simulink model "quad_control_sim_q"  (R2013a)
settings: Solver=ode3  StartTime=0.0  StopTime=5  FixedStep=0.005  RelTol=1e-3
values from neighbouring files (symbols this model uses):
  initial_states = [0;0;0;0;0;0;q0_init;0;q1_init;0;q2_init;0;q3_init;0]    [quad_control_sim_script_q.m]
  inputs = [x_accel_ref; y_accel_ref; a_u]    [quad_control_sim_script_q.m]
  params = [m;g;l;Jxx;Jyy;Jzz;k1;k2;k3;k4;b1;b2;b3;b4; d]    [quad_control_sim_script_q.m]
  pq = 1.2    [quad_control_sim_script_q.m]
  pw = 18    [quad_control_sim_script_q.m]
settings Model: Creator=Ken Katagiri  LastModifiedBy=Ken Katagiri

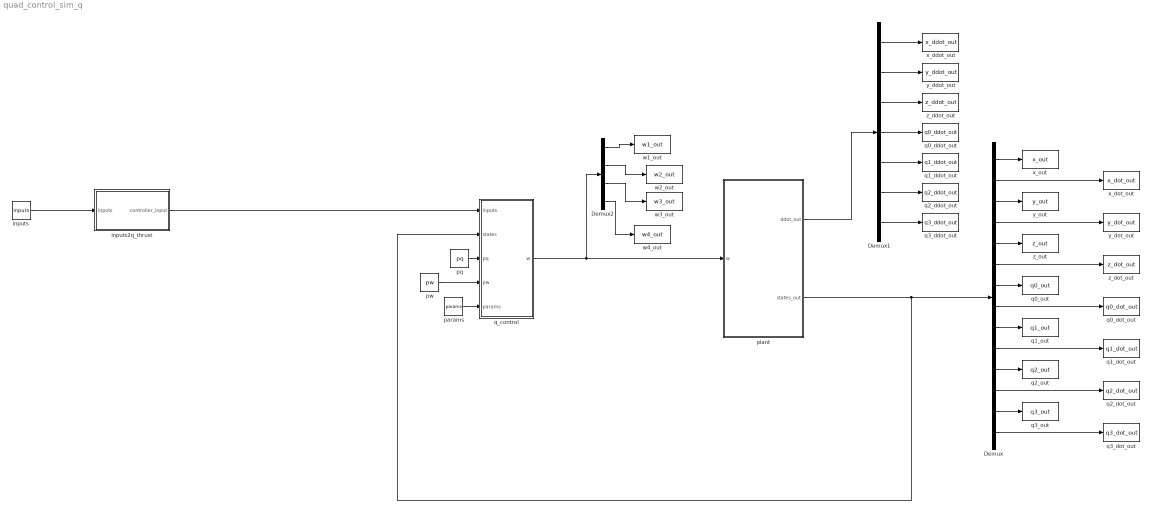
== system quad_control_sim_q ==
  Demux : Demux  Outputs=14
  Demux1 : Demux  Outputs=7
  Demux2 : Demux
  inputs : Constant  Value=inputs
  inputs2q_thrust : MATLAB Function  TreatAsAtomicUnit=on
  params : Constant  Value=params
  plant : Subsystem
  pq : Constant  Value=pq
  pw : Constant  Value=pw
  q0_ddot_out : ToWorkspace  VariableName=q0_ddot_out  SampleTime=-1
  q0_dot_out : ToWorkspace  VariableName=q0_dot_out  SampleTime=-1
  q0_out : ToWorkspace  VariableName=q0_out  SampleTime=-1
  q1_ddot_out : ToWorkspace  VariableName=q1_ddot_out  SampleTime=-1
  q1_dot_out : ToWorkspace  VariableName=q1_dot_out  SampleTime=-1
  q1_out : ToWorkspace  VariableName=q1_out  SampleTime=-1
  q2_ddot_out : ToWorkspace  VariableName=q2_ddot_out  SampleTime=-1
  q2_dot_out : ToWorkspace  VariableName=q2_dot_out  SampleTime=-1
  q2_out : ToWorkspace  VariableName=q2_out  SampleTime=-1
  q3_ddot_out : ToWorkspace  VariableName=q3_ddot_out  SampleTime=-1
  q3_dot_out : ToWorkspace  VariableName=q3_dot_out  SampleTime=-1
  q3_out : ToWorkspace  VariableName=q3_out  SampleTime=-1
  q_control : MATLAB Function  TreatAsAtomicUnit=on
  w1_out : ToWorkspace  VariableName=w1_out  SampleTime=-1
  w2_out : ToWorkspace  VariableName=w2_out  SampleTime=-1
  w3_out : ToWorkspace  VariableName=w3_out  SampleTime=-1
  w4_out : ToWorkspace  VariableName=w4_out  SampleTime=-1
  x_ddot_out : ToWorkspace  VariableName=x_ddot_out  SampleTime=-1
  x_dot_out : ToWorkspace  VariableName=x_dot_out  SampleTime=-1
  x_out : ToWorkspace  VariableName=x_out  SampleTime=-1
  y_ddot_out : ToWorkspace  VariableName=y_ddot_out  SampleTime=-1
  y_dot_out : ToWorkspace  VariableName=y_dot_out  SampleTime=-1
  y_out : ToWorkspace  VariableName=y_out  SampleTime=-1
  z_ddot_out : ToWorkspace  VariableName=z_ddot_out  SampleTime=-1
  z_dot_out : ToWorkspace  VariableName=z_dot_out  SampleTime=-1
  z_out : ToWorkspace  VariableName=z_out  SampleTime=-1
  wires:
  Demux/1 -> x_out/1
  Demux/3 -> y_out/1
  Demux/5 -> z_out/1
  Demux/7 -> q0_out/1
  Demux/9 -> q1_out/1
  Demux/11 -> q2_out/1
  Demux/13 -> q3_out/1
  Demux/2 -> x_dot_out/1
  Demux/4 -> y_dot_out/1
  Demux/6 -> z_dot_out/1
  Demux/8 -> q0_dot_out/1
  Demux/10 -> q1_dot_out/1
  Demux/12 -> q2_dot_out/1
  Demux/14 -> q3_dot_out/1
  Demux1/1 -> x_ddot_out/1
  Demux1/2 -> y_ddot_out/1
  Demux1/3 -> z_ddot_out/1
  Demux1/4 -> q0_ddot_out/1
  Demux1/5 -> q1_ddot_out/1
  Demux1/6 -> q2_ddot_out/1
  Demux1/7 -> q3_ddot_out/1
  plant/1(ddot_out) -> Demux1/1
  params/1 -> q_control/5(params)
  pq/1 -> q_control/3(pq)
  plant/2(states_out) -> q_control/2(states), Demux/1
  pw/1 -> q_control/4(pw)
  inputs/1 -> inputs2q_thrust/1(inputs)
  inputs2q_thrust/1(controller_input) -> q_control/1(inputs)
  q_control/1(w) -> Demux2/1, plant/1(w)
  Demux2/1 -> w1_out/1
  Demux2/2 -> w2_out/1
  Demux2/3 -> w3_out/1
  Demux2/4 -> w4_out/1

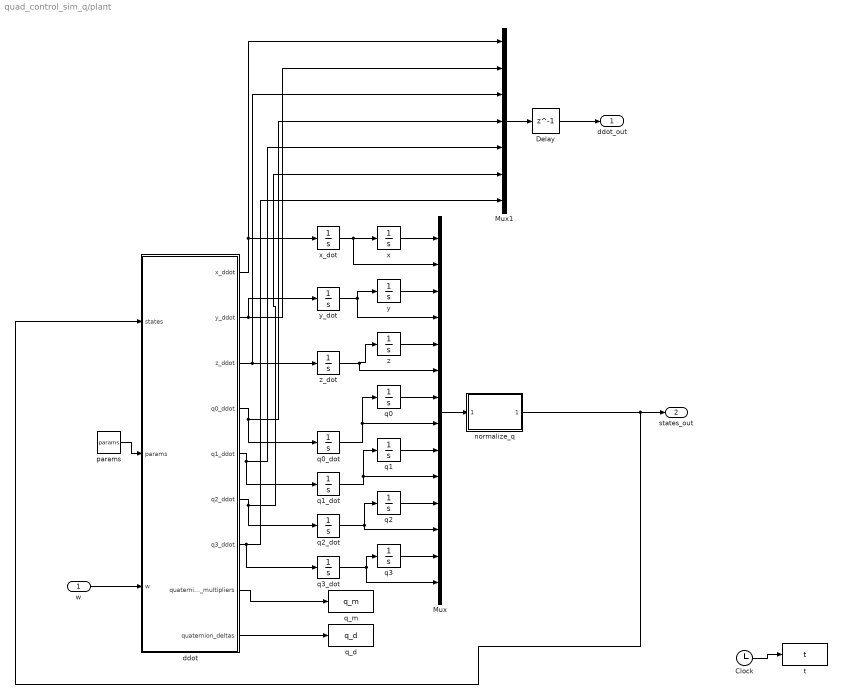
== system quad_control_sim_q/plant ==
  w : Inport
  Clock : Clock
  Delay : Delay  DelayLength=1  InitialCondition=[0; 0; 0; 0; 0; 0; 0]
  Mux : Mux  Inputs=14
  Mux1 : Mux  Inputs=7
  ddot : MATLAB Function  TreatAsAtomicUnit=on
  normalize_q : MATLAB Function  TreatAsAtomicUnit=on
  params : Constant  Value=params
  q0 : Integrator  InitialCondition=initial_states(7)
  q0_dot : Integrator
  q1 : Integrator  InitialCondition=initial_states(9)
  q1_dot : Integrator
  q2 : Integrator  InitialCondition=initial_states(11)
  q2_dot : Integrator
  q3 : Integrator  InitialCondition=initial_states(13)
  q3_dot : Integrator
  q_d : ToWorkspace  VariableName=q_d  SampleTime=-1
  q_m : ToWorkspace  VariableName=q_m  SampleTime=-1
  t : ToWorkspace  VariableName=t  SampleTime=-1
  x : Integrator  InitialCondition=initial_states(1)
  x_dot : Integrator
  y : Integrator  InitialCondition=initial_states(2)
  y_dot : Integrator
  z : Integrator  InitialCondition=initial_states(3)
  z_dot : Integrator
  ddot_out : Outport
  states_out : Outport  Port=2
  wires:
  ddot/7(q3_ddot) -> q3_dot/1, Mux1/7
  ddot/6(q2_ddot) -> Mux1/6, q2_dot/1
  ddot/5(q1_ddot) -> Mux1/5, q1_dot/1
  ddot/1(x_ddot) -> Mux1/1, x_dot/1
  ddot/2(y_ddot) -> Mux1/2, y_dot/1
  ddot/3(z_ddot) -> Mux1/3, z_dot/1
  ddot/4(q0_ddot) -> Mux1/4, q0_dot/1
  x_dot/1 -> Mux/2, x/1
  y_dot/1 -> Mux/4, y/1
  q3_dot/1 -> Mux/14, q3/1
  q2_dot/1 -> Mux/12, q2/1
  q1_dot/1 -> Mux/10, q1/1
  q0_dot/1 -> Mux/8, q0/1
  x/1 -> Mux/1
  y/1 -> Mux/3
  z/1 -> Mux/5
  z_dot/1 -> Mux/6, z/1
  q0/1 -> Mux/7
  q1/1 -> Mux/9
  q2/1 -> Mux/11
  q3/1 -> Mux/13
  params/1 -> ddot/2(params)
  Clock/1 -> t/1
  w/1 -> ddot/3(w)
  ddot/8(quaternion_multipliers) -> q_m/1
  ddot/9(quaternion_deltas) -> q_d/1
  Mux/1 -> normalize_q/1(states_in)
  normalize_q/1(states_out) -> states_out/1, ddot/1(states)
  Mux1/1 -> Delay/1
  Delay/1 -> ddot_out/1

== matlab function quad_control_sim_q/plant/normalize_q ==
  data: states_in input size=14; states_out output
function states_out = fcn(states_in)
%#codegen
    q0_in = states_in(7); q1_in = states_in(9); q2_in = states_in(11); q3_in = states_in(13);
    q_norm = norm([q0_in, q1_in, q2_in, q3_in]);
    q0_out = q0_in/q_norm; q1_out = q1_in/q_norm; q2_out = q2_in/q_norm; q3_out = q3_in/q_norm; 
    states_out = [states_in(1); states_in(2); states_in(3); states_in(4); states_in(5); states_in(6); ...
            q0_out; states_in(8); q1_out; states_in(10); q2_out; states_in(12); q3_out; states_in(14)];

== matlab function quad_control_sim_q/plant/ddot ==
  data: states input size=14; x_ddot output; y_ddot output; z_ddot output; q0_ddot output; q1_ddot output; q2_ddot output; q3_ddot output; params input; w input; quaternion_multipliers output; quaternion_deltas output
function [x_ddot, y_ddot, z_ddot, q0_ddot, q1_ddot, q2_ddot, q3_ddot, quaternion_multipliers, quaternion_deltas]= ddot(states, params, w)
%#codegen    
    m=params(1);
    g=params(2);
    l=params(3);

    Jxx=params(4);
    Jyy=params(5);
    Jzz=params(6);

    k1 = params(7);
    k2 = params(8);
    k3 = params(9);
    k4 = params(10);

    b1 = params(11);
    b2 = params(12);
    b3 = params(13);
    b4 = params(14);
    
    d = params(15);

    w1 = w(1);
    w2 = w(2);
    w3 = w(3);
    w4 = w(4);
    
    x = states(1); x_dot = states(2); y = states(3); y_dot = states(4); z = states(5); z_dot = states(6);

    q0 = states(7); q0_dot = states(8); q1 = states(9); q1_dot = states(10);
    q2 = states(11); q2_dot = states(12); q3 = states(13); q3_dot = states(14);
    
    upphi_x = 2*(k1*w1^2+k2*w2^2+k3*w3^2+k4*w4^2)*(q2*q0+q1*q3) ...
                + (-b1*w1^2+b2*w2^2+b3*w3^2-b4*w4^2)*(1-2*(q2^2+q3^2)) ...
                + 2*(b1*w1^2+b2*w2^2-b3*w3^2-b4*w4^2)*(q1*q2-q3*q0) - d*x_dot;
            
    upphi_y = 2*(k1*w1^2+k2*w2^2+k3*w3^2+k4*w4^2)*(q3*q2-q1*q0) ...
                + 2*(-b1*w1^2+b2*w2^2+b3*w3^2-b4*w4^2)*(q3*q0+q1*q2) ...
                + (b1*w1^2+b2*w2^2-b3*w3^2-b4*w4^2)*(1-2*(q1^2+q3^2)) - d*y_dot;
            
    upphi_z = (k1*w1^2+k2*w2^2+k3*w3^2+k4*w4^2)*(1-2*(q1^2+q2^2)) ...
                + 2*(-b1*w1^2+b2*w2^2+b3*w3^2-b4*w4^2)*(q3*q1-q2*q0) ...
                + 2*(b1*w1^2+b2*w2^2-b3*w3^2-b4*w4^2)*(q1*q0+q3*q2) - d*z_dot;
            
    T_e2E = [1-2*(q2^2+q3^2), 2*(q1*q2-q3*q0), 2*(q2*q0+q1*q3);
            2*(q3*q0+q1*q2), 1-2*(q1^2+q3^2), 2*(q3*q2-q1*q0);
            2*(q3*q1-q2*q0), 2*(q1*q0+q3*q2), 1-2*(q1^2+q2^2)];

            
    force_mult_1 = [-b1*w1^2-b3*w3^2; b1*w1^2+b3*w3^2; k1*w1^2-k3*w3^2];
    force_mult_2 = [b2*w2^2+b4*w4^2; b2*w2^2+b4*w4^2; k2*w2^2-k4*w4^2];
        
    force_mult_1_E = T_e2E*force_mult_1;
    force_mult_2_E = T_e2E*force_mult_2;
        
    dx1_dq0 = (l/sqrt(2))*[-2*q3; 2*q3; 2*q1-2*q2];
    dx2_dq0 = (l/sqrt(2))*[-2*q3; -2*q3; 2*q1+2*q2];
    upphi_q0 = dot(force_mult_1_E, dx1_dq0) + dot(force_mult_2_E, dx2_dq0);
    
    dx1_dq1 = (l/sqrt(2))*[2*q2; 2*q2-4*q1; 2*q0+2*q3];
    dx2_dq1 = (l/sqrt(2))*[2*q2; -4*q1-2*q2; 2*q0-2*q3];
    upphi_q1 = dot(force_mult_1_E, dx1_dq1) + dot(force_mult_2_E, dx2_dq1);
        
    dx1_dq2 = (l/sqrt(2))*[2*q1-4*q2; 2*q1; 2*q3-2*q0];
    dx2_dq2 = (l/sqrt(2))*[2*q1+4*q2; -2*q1; 2*q3+2*q0];
    upphi_q2 = dot(force_mult_1_E, dx1_dq2) + dot(force_mult_2_E, dx2_dq2);
    
    dx1_dq3 = (l/sqrt(2))*[-2*q0-4*q3; 2*q0-4*q3; 2*q1+2*q2];
    dx2_dq3 = (l/sqrt(2))*[-2*q0+4*q3; -4*q3-2*q0; 2*q2-2*q1];
    upphi_q3 = dot(force_mult_1_E, dx1_dq3) + dot(force_mult_2_E, dx2_dq3);
    
        
    delta1 = upphi_x;

    delta2 = upphi_y;

    delta3 = upphi_z;


    delta4 = upphi_q0 ...
                -8*Jxx*q0_dot*q1_dot*q1-8*Jyy*q0_dot*q2_dot*q2-8*Jzz*q0_dot*q3_dot*q3 ...
                +8*Jxx*q1_dot^2*q0+8*Jyy*q2_dot^2*q0+8*Jzz*q3_dot^2*q0 ...
                +(8*Jxx-8*Jyy)*q1_dot*q2_dot*q3+(8*Jzz-8*Jxx)*q1_dot*q3_dot*q2+(8*Jyy-8*Jzz)*q2_dot*q3_dot*q1;

    delta5 = upphi_q1 ...
                -8*Jxx*q0_dot*q1_dot*q0-8*Jyy*q1_dot*q3_dot*q3-8*Jzz*q1_dot*q2_dot*q2 ...
                +(8*Jyy-8*Jzz)*q2_dot*q3_dot*q0+(8*Jxx-8*Jyy)*q0_dot*q3_dot*q2+(8*Jzz-8*Jxx)*q0_dot*q2_dot*q3 ...
                +8*Jxx*q0_dot^2*q1+8*Jyy*q3_dot^2*q1+8*Jzz*q2_dot^2*q1;

    delta6 = upphi_q2 ...
                -8*Jxx*q2_dot*q3_dot*q3-8*Jyy*q0_dot*q2_dot*q0-8*Jzz*q1_dot*q2_dot*q1 ...
                +8*Jxx*q3_dot^2*q2+8*Jyy*q0_dot^2*q2+8*Jzz*q1_dot^2*q2 ...
                +8*(Jxx-Jyy)*q0_dot*q3_dot*q1+8*(Jyy-Jzz)*q0_dot*q1_dot*q3+8*(Jzz-Jxx)*q1_dot*q3_dot*q0;

    delta7 = upphi_q3 ...
                -8*Jxx*q2_dot*q3_dot*q2-8*Jyy*q1_dot*q3_dot*q1-8*Jzz*q0_dot*q3_dot*q0 ...
                +8*Jxx*q2_dot^2*q3+8*Jyy*q1_dot^2*q3+8*Jzz*q0_dot^2*q3 ...
                +(8*Jzz-8*Jxx)*q0_dot*q2_dot*q1+(8*Jxx-8*Jyy)*q1_dot*q2_dot*q0+(8*Jyy-8*Jzz)*q0_dot*q1_dot*q2;
            

    quaternion_deltas = [delta4; delta5; delta6; delta7; -q0_dot^2-q1_dot^2-q2_dot^2-q3_dot^2];

    quaternion_multipliers = ...
        [4*Jxx*q1^2+4*Jyy*q2^2+4*Jzz*q3^2, -4*Jzz*q2*q3+4*Jyy*q2*q3-4*Jxx*q0*q1, -4*Jxx*q1*q3+4*Jzz*q1*q3-4*Jyy*q0*q2, -4*Jyy*q1*q2+4*Jxx*q1*q2-4*Jzz*q0*q3;
         -4*Jzz*q2*q3+4*Jyy*q2*q3-4*Jxx*q0*q1, 4*Jxx*q0^2+4*Jyy*q3^2+4*Jzz*q2^2, -4*Jyy*q0*q3+4*Jxx*q0*q3-4*Jzz*q1*q2, -4*Jxx*q0*q2+4*Jzz*q0*q2-4*Jyy*q1*q3;
         -4*Jxx*q1*q3+4*Jzz*q1*q3-4*Jyy*q0*q2, -4*Jyy*q0*q3+4*Jxx*q0*q3-4*Jzz*q1*q2, 4*Jxx*q3^2+4*Jyy*q0^2+4*Jzz*q1^2, -4*Jzz*q0*q1+4*Jyy*q0*q1-4*Jxx*q2*q3;
         -4*Jyy*q1*q2+4*Jxx*q1*q2-4*Jzz*q0*q3, -4*Jxx*q0*q2+4*Jzz*q0*q2-4*Jyy*q1*q3, -4*Jzz*q0*q1+4*Jyy*q0*q1-4*Jxx*q2*q3, 4*Jxx*q2^2+4*Jyy*q1^2+4*Jzz*q0^2;
         q0, q1, q2, q3];

    q_ddot = quaternion_multipliers\quaternion_deltas;

    
    
    
    x_ddot = delta1/m;
    y_ddot = delta2/m;
    z_ddot= delta3/m-g;  
    q0_ddot = q_ddot(1);
    q1_ddot = q_ddot(2);
    q2_ddot = q_ddot(3);
    q3_ddot = q_ddot(4);

== matlab function quad_control_sim_q/q_control ==
  data: inputs input; states input; w output size=4; pq input; pw input; params input
function w = fcn(inputs, states, pq, pw, params)

    m=params(1);
    g=params(2);
    l=params(3);

    Jxx=params(4);
    Jyy=params(5);
    Jzz=params(6);

    k1 = params(7);
    k2 = params(8);
    k3 = params(9);
    k4 = params(10);

    b1 = params(11);
    b2 = params(12);
    b3 = params(13);
    b4 = params(14);
    
    d = params(15);
    
    q0=states(7); q1=states(9); q2=states(11); q3=states(13);
    q0_dot=states(8); q1_dot=states(10); q2_dot=states(12); q3_dot=states(14);

    q0_r = inputs(1); q1_r = inputs(2); q2_r = inputs(3); q3_r = inputs(4); a_u = inputs(5);
    
    q0_err = q0_r*q0+q1_r*q1+q2_r*q2+q3_r*q3;
    q1_err = q1_r*q0+q3_r*q2-q0_r*q1-q3_r*q3;
    q2_err = q2_r*q0+q1_r*q3-q3_r*q1-q0_r*q2;
    q3_err = q3_r*q0+q2_r*q1-q1_r*q2-q0_r*q3;
    
    if q0_err < 0
        q1_err = -q1_err;
        q2_err = -q2_err;
        q3_err = -q3_err;
    end

    %%%%%%%%%%%%NORMALIZE ERROR QUATERNION
    n = norm([q0_err; q1_err; q2_err; q3_err]);
    q0_err = q0_err/n; q1_err = q1_err/n; q2_err = q2_err/n; q3_err = q3_err/n; 
    
    wx = 2*(q1_dot*q0+q2_dot*q3-q3_dot*q2-q0_dot*q1);
    wy = 2*(q3_dot*q1+q2_dot*q0-q1_dot*q3-q0_dot*q2);
    wz = 2*(q3_dot*q0+q1_dot*q2-q2_dot*q1-q0_dot*q3);
    
    
    %disp('------------');

    tau_x = pq*q1_err-pw*Jxx*(l/sqrt(2))*wx;
    tau_y = pq*q2_err-pw*Jyy*(l/sqrt(2))*wy;
    tau_z = pq*q3_err-pw*Jzz*l*(wz);

    gamma1 = (sqrt(2)/l)*tau_x;
    gamma2 = (sqrt(2)/l)*tau_y;
    gamma3 = (m*a_u)/(cos(2*acos(q0)));
    gamma4 = (1/l)*tau_z;
    

    w3_sq3 = (gamma4+(b1/k1)*((gamma2-gamma1)/2)+(b2/k2)*((gamma2+gamma3)/2)+(b4/k4)*((gamma3-gamma1)/2))/((b1/k1)*k3+(b2/k2)*k3+b3+(b4/k4)*k3);
    w1_sq3 = ((gamma1-gamma2)/2+k3*w3_sq3)/k1;
    w2_sq3 = ((gamma2+gamma3)/2-k3*w3_sq3)/k2;
    w4_sq3 = ((gamma3-gamma1)/2-k3*w3_sq3)/k4;
    
    w2_sq = ((b1/k1)*((gamma1+gamma3)/2)+(b3/k3)*((gamma2+gamma3)/2)+(b4/k4)*((gamma1+gamma2)/2)-gamma4)/((b1/k1)*k2+b2+(b3/k3)*k2+(b4/k4)*k2);
    w1_sq = ((gamma1+gamma3)/2-k2*w2_sq)/k1;
    w3_sq = ((gamma2+gamma3)/2-k2*w2_sq)/k3;
    w4_sq = (k2*w2_sq-(gamma1+gamma2)/2)/k4;

    w1 = sqrt(max(0, w1_sq));
    w2 = sqrt(max(0, w2_sq));
    w3 = sqrt(max(0, w3_sq));
    w4 = sqrt(max(0, w4_sq));
        
    w = [w1; w2; w3; w4];

== matlab function quad_control_sim_q/inputs2q_thrust ==
  data: inputs input; controller_input output
function controller_input = fcn(inputs)
%#codegen
    x_accel_multiplier = inputs(1);
    y_accel_multiplier = inputs(2);
    
    del = x_accel_multiplier*0.01;
    ep = y_accel_multiplier*0.01;
    
    q0 = cos(del)*cos(ep);
    q1 = -cos(del)*sin(ep);
    q2 = sin(del)*cos(ep);
    q3 = sin(del)*sin(ep);
    
    controller_input = [q0; q1; q2; q3; inputs(3)];
